simulink subsystem "EnvTrig"  (R2024a)
settings: Solver=VariableStepAuto  StartTime=0.0  StopTime=10.0  RelTol=1e-3
settings Model: Creator=dfurodet  LastModifiedBy=dfurodet

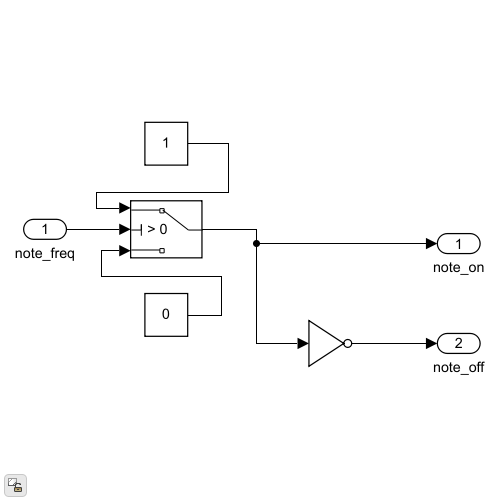
[thumbnail: Simulink's stored preview of the top-level diagram]
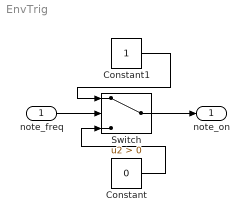
== system EnvTrig ==
  note_freq : Inport
  Constant : Constant  Value=0  OutDataTypeStr=boolean
  Constant1 : Constant  OutDataTypeStr=boolean
  Switch : Switch  Criteria=u2 > Threshold  SaturateOnIntegerOverflow=off  InputSameDT=off
  note_on : Outport
  wires:
  note_freq/1 -> Switch/2
  Switch/1 -> note_on/1
  Constant1/1 -> Switch/1
  Constant/1 -> Switch/3
